simulink model "spring"  (R2018b)
settings: Solver=VariableStepAuto  StartTime=0.0  StopTime=10.0  RelTol=1e-3
values from neighbouring files (symbols this model uses):
  B = 12    [codespring.m]
  F = 8    [codespring.m]
  K = 16    [codespring.m]
  M = 2    [codespring.m]
  x0 = 4    [codespring.m]
settings Model: Creator=student  LastModifiedBy=student

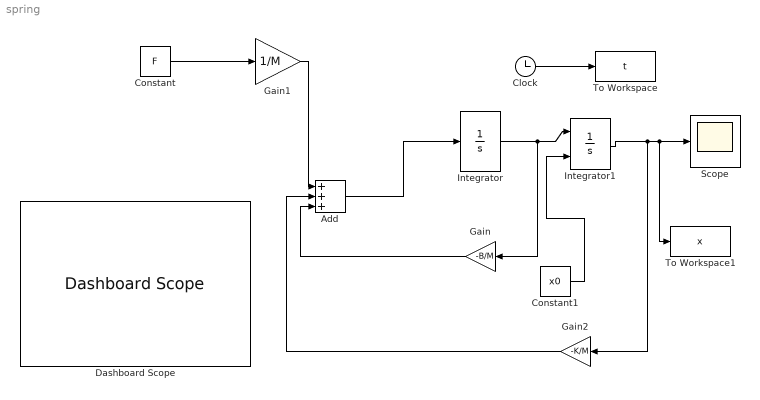
== system spring ==
  Add : Sum  Inputs=+++
  Clock : Clock
  Constant : Constant  Value=F
  Constant1 : Constant  Value=x0
  Dashboard Scope : DashboardScope  WebBlockId=13
  Gain : Gain  Gain=-B/M
  Gain1 : Gain  Gain=1/M
  Gain2 : Gain  Gain=-K/M
  Integrator : Integrator
  Integrator1 : Integrator  InitialConditionSource=external
  Scope : Scope
  To Workspace : ToWorkspace  VariableName=t  SaveFormat=Timeseries  SampleTime=-1
  To Workspace1 : ToWorkspace  VariableName=x  SampleTime=-1
  wires:
  Integrator/1 -> Gain/1, Integrator1/1
  Integrator1/1 -> Gain2/1, To Workspace1/1, Scope/1
  Constant/1 -> Gain1/1
  Add/1 -> Integrator/1
  Gain1/1 -> Add/1
  Gain/1 -> Add/3
  Gain2/1 -> Add/2
  Clock/1 -> To Workspace/1
  Constant1/1 -> Integrator1/2
